simulink model "Part2_FSK"  (R2017a)
settings: Solver=VariableStepAuto  StartTime=0.0  StopTime=1  RelTol=1e-3
undefined symbols (not defined in the file): randseed
libraries: commrandsrc3 x1, commfilt2 x1
settings Model: Creator=Marine  LastModifiedBy=mhuynh7
settings SFSimCC: SimUseLocalCustomCode=on
settings RTWCC: RTWUseLocalCustomCode=on

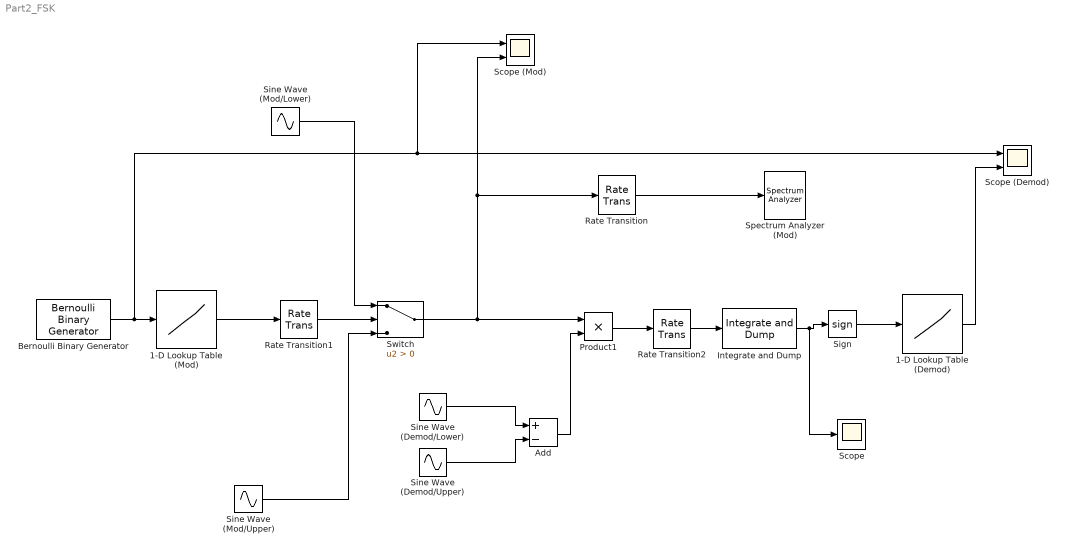
== system Part2_FSK ==
  1-D Lookup Table (Demod) : Lookup_n-D  NumberOfTableDimensions=1  BreakpointsForDimension1=[-1,0,1]  Table=[0,0,1]  InternalRulePriority=Speed  RndMeth=Simplest  InputSameDT=on
  1-D Lookup Table (Mod) : Lookup_n-D  NumberOfTableDimensions=1  BreakpointsForDimension1=[0,1]  Table=[-1,1]  InternalRulePriority=Speed  RndMeth=Simplest  InputSameDT=on
  Add : Sum  Inputs=+-
  Bernoulli Binary Generator : commrandsrc3/Bernoulli Binary Generator  ProbabilityOfZero=0.5  SeedSource=Parameter  Seed=randseed  SampleTime=0.001  SamplesPerFrame=1  OutputDataType=double  SimulateUsing=Interpreted execution
  Integrate and Dump : commfilt2/Integrate and Dump  obssamples=8  offsetsamples=0  nodump=off  roundingMode=Floor  overflowMode=off  outputDataTypeStr=Inherit: Same as accumulator  outputLastDataTypeStr=Inherit: Same as accumulator
      settings: SourceProductName=Communications System Toolbox
  Product1 : Product
  Rate Transition : RateTransition  OutPortSampleTime=0.5e-4
  Rate Transition1 : RateTransition  OutPortSampleTime=0.5e-4
  Rate Transition2 : RateTransition  OutPortSampleTime=0.5e-4
  Scope : Scope
  Scope (Demod) : Scope  NumInputPorts=2
  Scope (Mod) : Scope  NumInputPorts=2
  Sign : Signum
  Sine Wave (Demod/Lower) : Sin  SineType=Sample based  Samples=4000  SampleTime=1e-7
  Sine Wave (Demod/Upper) : Sin  SineType=Sample based  Samples=2857  SampleTime=1e-7
  Sine Wave (Mod/Lower) : Sin  SineType=Sample based  Samples=4000  SampleTime=1e-7
  Sine Wave (Mod/Upper) : Sin  SineType=Sample based  Samples=2857  SampleTime=1e-7
  Spectrum Analyzer (Mod) : SpectrumAnalyzer
  Switch : Switch  Criteria=u2 > Threshold
  wires:
  Sine Wave (Mod/Upper)/1 -> Switch/3
  Switch/1 -> Scope (Mod)/2, Rate Transition/1, Product1/1
  Rate Transition/1 -> Spectrum Analyzer (Mod)/1
  1-D Lookup Table (Demod)/1 -> Scope (Demod)/2
  Sign/1 -> 1-D Lookup Table (Demod)/1
  1-D Lookup Table (Mod)/1 -> Rate Transition1/1
  Rate Transition1/1 -> Switch/2
  Sine Wave (Mod/Lower)/1 -> Switch/1
  Sine Wave (Demod/Lower)/1 -> Add/1
  Sine Wave (Demod/Upper)/1 -> Add/2
  Add/1 -> Product1/2
  Product1/1 -> Rate Transition2/1
  Bernoulli Binary Generator/1 -> Scope (Mod)/1, Scope (Demod)/1, 1-D Lookup Table (Mod)/1
  Rate Transition2/1 -> Integrate and Dump/1
  Integrate and Dump/1 -> Scope/1, Sign/1
